simulink model "trajectory_optimization"  (R2014a)
settings: Solver=FixedStepDiscrete  StartTime=0.0  StopTime=inf  FixedStep=sample_time  RelTol=1e-3
undefined symbols (not defined in the file): alpha_apex, boom_mount_angle, control_start_time, d_y_boom_com_offset, d_y_boom_hip_offset, d_y_com, d_y_mount_to_com, DiscIntNeverNeededParam, g, h_boom, i_limit_lateral, j_segments, kd_angle, kd_lateral, kd_length, kd_motor, ki_lateral, kp_angle, kp_lateral, kp_length, kp_motor, l0_virtual, l_boom, l_boom_projected, l_retract_swing, l_seg, lateral_offset, m_leg_motor, magnitude, max_back_bar_angle, max_front_bar_angle, max_leg_angle, max_leg_length, max_torque_lateral, min_back_bar_angle, min_front_bar_angle, min_leg_angle, min_leg_length, reset_leg_angle, reset_leg_length, run_trajectory, sample_time, sea_coulomb_friction, sea_offset_friction, secondary_to_apex_target, time_to_apex, velocity_avg_samples
libraries: simulink x5
(part 1 of 2)
settings Model: xpc_rtwmakecfg_data=_xpcethercatlib_  BufferReuse=off  Creator=wmartin  LastModifiedBy=wmartin
settings SolverCC: EnableConcurrentExecution=on
settings DataIOCC: MaxDataPoints=1000000000  SaveFormat=StructureWithTime
settings OptimizationCC: BlockReduction=off  OptimizeBlockIOStorage=off  BufferReuse=off  GlobalBufferReuse=off  ExpressionFolding=off  ExpressionDepthLimit=2147483647  LocalBlockOutputs=off  SimCompilerOptimization=On
settings DebuggingCC: UnderspecifiedInitializationDetection=Classic  StateNameClashWarn=warning
settings HardwareCC: ProdIntDivRoundTo=Zero  ProdEndianess=LittleEndian  ProdHWDeviceType=Generic->32-bit x86 compatible
settings ModelReferenceCC: UpdateModelReferenceTargets=IfOutOfDate  EnableParallelModelReferenceBuilds=on  ParallelModelReferenceMATLABWorkerInit=Copy Base Workspace
settings RTWCC: SystemTargetFile=slrt.tlc  TemplateMakefile=slrt_default_tmf  Description=Simulink Real-Time  RTWVerbose=off  ProcessScript=slrt_make_rtw_hook  RTWCompilerOptimization=On
settings CodeAppCC: MaxIdLength=127
settings SimulinkRealTimeCC: GeneratePreprocessorConditionals=Disable all  EnableShiftOperators=on  RL32LogBufSizeModifier=100000000

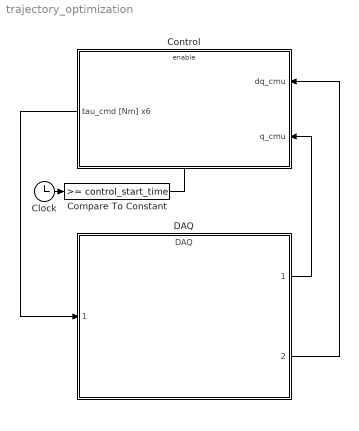
== system trajectory_optimization ==
  Clock : Clock
  Compare To Constant : simulink/Logic and Bit Operations/Compare To Constant  relop=>=  const=control_start_time  OutDataTypeStr=boolean
  Control : Subsystem
  DAQ : ModelReference  ModelNameDialog=DAQ  SimulationMode=Normal  ModelReferenceVersion=1.1653  CopyOfModelName=DAQ  DefaultDataLogging=on
  wires:
  DAQ/1 -> Control/2(q_cmu)
  DAQ/2 -> Control/1(dq_cmu)
  Clock/1 -> Compare To Constant/1
  Compare To Constant/1 -> Control/Enable
  Control/1(tau_cmd [Nm] x6) -> DAQ/1

== system trajectory_optimization/Control ==
  dq_cmu : Inport
  q_cmu : Inport  Port=2
  Enable : EnablePort  StatesWhenEnabling=reset
  Actuator Control : ModelReference  ModelNameDialog=Actuator_Control  SimulationMode=Normal  ModelReferenceVersion=1.16  CopyOfModelName=Actuator_Control  DefaultDataLogging=on
  Behavior Control : Subsystem
  Disable SEA Control : Constant  Value=[0 0 0 0]  OutDataTypeStr=boolean
  tau_cmd [Nm] x6 : Outport  InitialOutput=[0 0 0 0 0 0]
  wires:
  Behavior Control/1(motor_torque_cmd) -> Actuator Control/1
  dq_cmu/1 -> Actuator Control/4, Behavior Control/1(dq_cmu)
  Actuator Control/1 -> tau_cmd [Nm] x6/1
  q_cmu/1 -> Actuator Control/3, Behavior Control/2(q_cmu)
  Disable SEA Control/1 -> Actuator Control/2

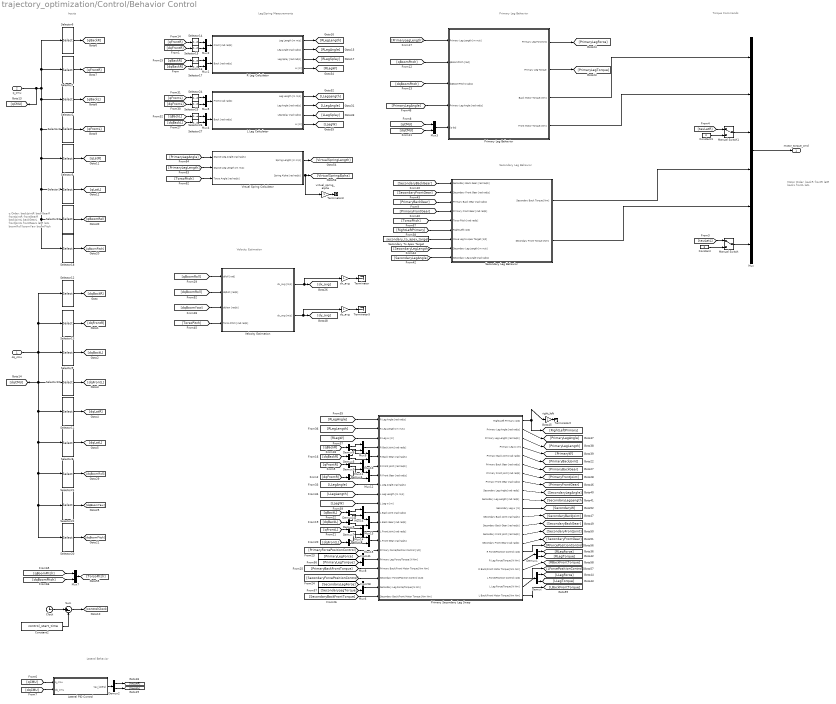
== system trajectory_optimization/Control/Behavior Control ==
  note: Motor Order:
      |
      | backR
      | frontR
      | latR
      | backL
      | frontL
      | latL
  note: q Order:
      |
      | backJointR
      | backGearR
      | frontJointR
      | frontGearR
      |
      | backJointL
      | backGearL
      | frontJointL
      | frontGearL
      |
      | latR
      | latL
      |
      | boomRoll
      | boomYaw
      | boomPitch
  note: Inputs
  note: Primary Leg Behavior
  note: Secondary Leg Behavior
  note: Torque Commands
  note: Lateral Behavior
  note: Leg/Spring Measurements
  note: Velocity Estimation
  dq_cmu : Inport
  q_cmu : Inport  Port=2
  Clock : Clock
  Constant : Constant  Value=0
  Constant1 : Constant  Value=0
  Constant2 : Constant  Value=control_start_time
  Demux{,1..10} (11 alike) : Demux  Outputs=2
  L Leg Calculator : Subsystem
  Lateral PID Control : Subsystem
  Manual Switch : ManualSwitch
  Manual Switch1 : ManualSwitch
  Mux : Mux  Inputs=6
  Mux{1..16} (16 alike) : Mux  Inputs=2
  Primary Leg Behavior : Subsystem
  Primary Secondary Leg Swap : Subsystem
  R Leg Calculator : Subsystem
  Secondary Leg Behavior : Subsystem
  Secondary To Apex Target : Constant  Value=secondary_to_apex_target  OutDataTypeStr=boolean
  Selector1 : Selector  InputPortWidth=13  Indices=[10]
  Selector10 : Selector  InputPortWidth=13  Indices=[7 8]
  Selector11 : Selector  InputPortWidth=13  Indices=[9]
  Selector12 : Selector  InputPortWidth=13  Indices=[1 2]
  Selector13 : Selector  InputPortWidth=13  Indices=[3 4]
  Selector{14..17,24..27} (8 alike) : Selector  InputPortWidth=2  Indices=[1]
  Selector18 : Selector  InputPortWidth=13  Indices=[13]
  Selector2 : Selector  InputPortWidth=13  Indices=[5 6]
  Selector20 : Selector  InputPortWidth=13  Indices=[13]
  Selector21 : Selector  InputPortWidth=13  Indices=[11]
  Selector22 : Selector  InputPortWidth=13  Indices=[12]
  Selector23 : Selector  InputPortWidth=13  Indices=[11]
  Selector4 : Selector  InputPortWidth=13  Indices=[7 8]
  Selector5 : Selector  InputPortWidth=13  Indices=[9]
  Selector6 : Selector  InputPortWidth=13  Indices=[1 2]
  Selector7 : Selector  InputPortWidth=13  Indices=[3 4]
  Selector8 : Selector  InputPortWidth=13  Indices=[10]
  Selector9 : Selector  InputPortWidth=13  Indices=[5 6]
  Sum : Sum  Inputs=|+-
  Terminator{,2..3,5} (4 alike) : Terminator
  Velocity Estimation : Subsystem
  Virtual Spring Calculator : Subsystem
  dx_avg : Gain
  dy_avg : Gain
  right_left : Gain
  virtual_spring_alpha : Gain
  motor_torque_cmd : Outport  OutputWhenDisabled=reset  InitialOutput=[0 0 0 0 0 0]
  wires:
  Lateral PID Control/1(tau_lateral) -> Demux2/1
  [dqCMU] -> Lateral PID Control/2(dq_cmu)
  [qCMU] -> Lateral PID Control/1(q_cmu)
  Sum/1 -> [controlClock]
  Selector4/1 -> [qFrontL]
  Selector2/1 -> [qBackL]
  Selector7/1 -> [qFrontR]
  Selector6/1 -> [qBackR]
  Selector1/1 -> [qLatL]
  Selector5/1 -> [qLatR]
  Constant2/1 -> Sum/2
  Clock/1 -> Sum/1
  Constant1/1 -> Manual Switch1/2
  Constant/1 -> Manual Switch/2
  Manual Switch/1 -> Mux/6
  Manual Switch1/1 -> Mux/3
  Mux/1 -> motor_torque_cmd/1
  Selector8/1 -> [dqLatL]
  Selector11/1 -> [dqLatR]
  Selector12/1 -> [dqBackR]
  Selector13/1 -> [dqFrontR]
  Selector9/1 -> [dqBackL]
  Selector10/1 -> [dqFrontL]
  [qBackR] -> Selector16/1
  [dqBackR] -> Selector17/1
  [qFrontR] -> Selector14/1
  [dqFrontR] -> Selector15/1
  Mux2/1 -> R Leg Calculator/1(Front [rad rad/s])
  Mux1/1 -> R Leg Calculator/2(Back [rad rad/s])
  R Leg Calculator/1("Leg Length [m m/s] ") -> [RLegLength]
  R Leg Calculator/2(Leg Angle [rad rad/s]) -> [RLegAngle]
  R Leg Calculator/3(Leg Splay [rad rad/s]) -> [RLegSplay]
  Demux2/1 -> [tauLatR]
  Demux2/2 -> [tauLatL]
  [tauLatR] -> Manual Switch1/1
  [tauLatL] -> Manual Switch/1
  Selector14/1 -> Mux2/1
  Selector15/1 -> Mux2/2
  Selector17/1 -> Mux1/2
  Selector16/1 -> Mux1/1
  q_cmu/1 -> Selector6/1, Selector7/1, Selector2/1, Selector4/1, Selector5/1, Selector18/1, Selector23/1, Selector1/1, [qCMU]
  Selector18/1 -> [qBoomPitch]
  Selector20/1 -> [dqBoomPitch]
  Selector22/1 -> [dqBoomYaw]
  dq_cmu/1 -> Selector20/1, Selector22/1, Selector21/1, Selector8/1, Selector11/1, Selector10/1, [dqCMU], Selector12/1, Selector13/1, Selector9/1
  Selector21/1 -> [dqBoomRoll]
  Selector23/1 -> [qBoomRoll]
  [qBackL] -> Selector26/1
  [dqBackL] -> Selector27/1
  [qFrontL] -> Selector24/1
  [dqFrontL] -> Selector25/1
  Mux5/1 -> L Leg Calculator/1(Front [rad rad/s])
  Mux4/1 -> L Leg Calculator/2(Back [rad rad/s])
  L Leg Calculator/1("Leg Length [m m/s] ") -> [LLegLength]
  L Leg Calculator/2(Leg Angle [rad rad/s]) -> [LLegAngle]
  L Leg Calculator/3(Leg Splay [rad rad/s]) -> [LLegSplay]
  Selector24/1 -> Mux5/1
  Selector25/1 -> Mux5/2
  Selector27/1 -> Mux4/2
  Selector26/1 -> Mux4/1
  R Leg Calculator/4(w [m]) -> [RLegW]
  L Leg Calculator/4(w [m]) -> [LLegW]
  Primary Secondary Leg Swap/1(Right/Left Primary [1/0]) -> right_left/1, [RightLeftPrimary]
  [PrimaryLegLength] -> Primary Leg Behavior/1(Primary Leg Length [m m/s])
  [qBoomPitch] -> Primary Leg Behavior/2(qBoomPitch [rad])
  [dqBoomPitch] -> Primary Leg Behavior/3(dqBoomPitch [rad/s])
  Primary Leg Behavior/1(Primary Leg Force [N]) -> [PrimaryLegForce]
  Primary Leg Behavior/2(Primary Leg Torque) -> [PrimaryLegTorque]
  Velocity Estimation/1(dx_avg [m/s]) -> dx_avg/1, [dx_avg]
  [qBoomRoll] -> Velocity Estimation/1(qRoll [rad])
  [dqBoomYaw] -> Velocity Estimation/3(dqYaw [rad/s])
  dx_avg/1 -> Terminator/1
  [PrimaryBackGear] -> Secondary Leg Behavior/3(Primary Back Gear [rad rad/s])
  [SecondaryBackGear] -> Secondary Leg Behavior/1(Secondary Back Gear [rad rad/s])
  [SecondaryFrontGear] -> Secondary Leg Behavior/2(Secondary Front Gear [rad rad/s])
  right_left/1 -> Terminator2/1
  Velocity Estimation/2(dy_avg [m/s]) -> dy_avg/1, [dy_avg]
  dy_avg/1 -> Terminator5/1
  [dqBoomRoll] -> Velocity Estimation/2(dqRoll [rad/s])
  [PrimaryLegAngle] -> Virtual Spring Calculator/1("Stance Leg Angle [rad rad/s] ")
  [PrimaryLegLength] -> Virtual Spring Calculator/2(Stance Leg Length [m m/s])
  Virtual Spring Calculator/1(Spring Length [m m/s]) -> [VirtualSpringLength]
  [TorsoPitch] -> Virtual Spring Calculator/3(Torso Angle [rad rad/s])
  Virtual Spring Calculator/2(Spring Alpha [rad rad/s]) -> virtual_spring_alpha/1, [VirtualSpringAlpha]
  [qBoomPitch] -> Mux7/1
  [dqBoomPitch] -> Mux7/2
  Mux7/1 -> [TorsoPitch]
  [TorsoPitch] -> Secondary Leg Behavior/5(Torso Pitch [rad rad/s])
  [TorsoPitch] -> Velocity Estimation/4(Torso Pitch [rad rad/s])
  [PrimaryLegAngle] -> Primary Leg Behavior/4(Primary Leg Angle [rad rad/s])
  virtual_spring_alpha/1 -> Terminator3/1
  Primary Leg Behavior/3(Back Motor Torque [Nm]) -> Mux/1
  Primary Leg Behavior/4(Front Motor Torque [Nm]) -> Mux/2
  [qCMU] -> Mux3/1
  [dqCMU] -> Mux3/2
  Mux3/1 -> Primary Leg Behavior/5("[q dq]")
  Secondary Leg Behavior/1(Secondary Back Torque [Nm]) -> Mux/4
  Secondary Leg Behavior/2(Secondary Front Torque [Nm]) -> Mux/5
  Primary Secondary Leg Swap/2(Primary Leg Angle [rad rad/s]) -> [PrimaryLegAngle]
  Primary Secondary Leg Swap/4(Primary Leg w [m]) -> [PrimaryW]
  Primary Secondary Leg Swap/3(Primary Leg Length [rad rad/s]) -> [PrimaryLegLength]
  [RLegAngle] -> Primary Secondary Leg Swap/1(R Leg Angle [rad rad/s])
  [RLegLength] -> Primary Secondary Leg Swap/2(R Leg Length [m m/s])
  [RLegW] -> Primary Secondary Leg Swap/3(R Leg w [m])
  [LLegAngle] -> Primary Secondary Leg Swap/8(L Leg Angle [rad rad/s])
  [LLegLength] -> Primary Secondary Leg Swap/9(L Leg Length [m m/s])
  [LLegW] -> Primary Secondary Leg Swap/10(L Leg w [m])
  [SecondaryLegForce] -> Mux6/1
  [SecondaryLegTorque] -> Mux6/2
  Mux6/1 -> Primary Secondary Leg Swap/19(Secondary Leg Force/Torque [N Nm])
  Mux8/1 -> Primary Secondary Leg Swap/16(Primary Leg Force/Torque [N Nm])
  [PrimaryLegTorque] -> Mux8/2
  [PrimaryLegForce] -> Mux8/1
  Primary Secondary Leg Swap/10(Secondary Leg Length [rad rad/s]) -> [SecondaryLegLength]
  Primary Secondary Leg Swap/9(Secondary Leg Angle [rad rad/s]) -> [SecondaryLegAngle]
  Primary Secondary Leg Swap/20(L Leg Force/Torque [N Nm]) -> Demux/1
  Demux/1 -> [LLegForce]
  Demux/2 -> [LLegTorque]
  Primary Secondary Leg Swap/17(R Leg Force/Torque [N Nm]) -> Demux1/1
  Demux1/1 -> [RLegForce]
  Demux1/2 -> [RLegTorque]
  [qFrontR] -> Demux3/1
  [dqFrontR] -> Demux4/1
  Mux9/1 -> Primary Secondary Leg Swap/4(R Back Joint [rad rad/s])
  Mux10/1 -> Primary Secondary Leg Swap/5(R Back Gear [rad rad/s])
  Mux11/1 -> Primary Secondary Leg Swap/6(R Front Joint [rad rad/s])
  Mux12/1 -> Primary Secondary Leg Swap/7(R Front Gear [rad rad/s])
  Demux3/1 -> Mux11/1
  Demux3/2 -> Mux12/1
  Demux4/1 -> Mux11/2
  Demux4/2 -> Mux12/2
  [dqBackR] -> Demux5/1
  [qBackR] -> Demux6/1
  Demux6/1 -> Mux9/1
  Demux6/2 -> Mux10/1
  Demux5/1 -> Mux9/2
  Demux5/2 -> Mux10/2
  [qFrontL] -> Demux7/1
  [dqFrontL] -> Demux8/1
  Mux16/1 -> Primary Secondary Leg Swap/11(L Back Joint [rad rad/s])
  Mux13/1 -> Primary Secondary Leg Swap/12(L Back Gear [rad rad/s])
  Mux14/1 -> Primary Secondary Leg Swap/13(L Front Joint [rad rad/s])
  Mux15/1 -> Primary Secondary Leg Swap/14(L Front Gear [rad rad/s])
  Demux7/1 -> Mux14/1
  Demux7/2 -> Mux15/1
  Demux8/1 -> Mux14/2
  Demux8/2 -> Mux15/2
  [dqBackL] -> Demux9/1
  [qBackL] -> Demux10/1
  Demux10/1 -> Mux16/1
  Demux10/2 -> Mux13/1
  Demux9/1 -> Mux16/2
  Demux9/2 -> Mux13/2
  [PrimaryForcePositionControl] -> Primary Secondary Leg Swap/15(Primary Force/Position Control [1/0])
  [SecondaryForcePositionControl] -> Primary Secondary Leg Swap/18(Secondary Force/Position Control [1/0])
  [PrimaryBackFrontTorque] -> Primary Secondary Leg Swap/17(Primary Back/Front Motor Torque [Nm Nm])
  [SecondaryBackFrontTorque] -> Primary Secondary Leg Swap/20(Secondary Back/Front Motor Torque [Nm Nm])
  Primary Secondary Leg Swap/5(Primary Back Joint [rad rad/s]) -> [PrimaryBackJoint]
  Primary Secondary Leg Swap/6(Primary Back Gear [rad rad/s]) -> [PrimaryBackGear]
  Primary Secondary Leg Swap/7(Primary Front Joint [rad rad/s]) -> [PrimaryFrontJoint]
  Primary Secondary Leg Swap/8(Primary Front Gear [rad rad/s]) -> [PrimaryFrontGear]
  Primary Secondary Leg Swap/12(Secondary Back Joint [rad rad/s]) -> [SecondaryBackJoint]
  Primary Secondary Leg Swap/13(Secondary Back Gear [rad rad/s]) -> [SecondaryBackGear]
  Primary Secondary Leg Swap/14(Secondary Front Joint [rad rad/s]) -> [SecondaryFrontJoint]
  Primary Secondary Leg Swap/15(Secondary Front Gear [rad rad/s]) -> [SecondaryFrontGear]
  Primary Secondary Leg Swap/11(Secondary Leg w [m]) -> [SecondaryW]
  Primary Secondary Leg Swap/19(L Force/Position Control [1/0]) -> [LForcePositionControl]
  Primary Secondary Leg Swap/16(R Force/Position Control [1/0]) -> [RForcePositionControl]
  Primary Secondary Leg Swap/18(R Back/Front Motor Torque [Nm Nm]) -> [RBackFrontTorque]
  Primary Secondary Leg Swap/21(L Back/Front Motor Torque [Nm Nm]) -> [LBackFrontTorque]
  [RightLeftPrimary] -> Secondary Leg Behavior/6(Right/Left [1/0])
  [PrimaryFrontGear] -> Secondary Leg Behavior/4(Primary Front Gear [rad rad/s])
  [SecondaryLegAngle] -> Secondary Leg Behavior/9(Secondary Leg Angle [rad rad/s])
  [SecondaryLegLength] -> Secondary Leg Behavior/8(Secondary Leg Length [m m/s])
  Secondary To Apex Target/1 -> Secondary Leg Behavior/7(Move Leg to Apex Target [1/0])

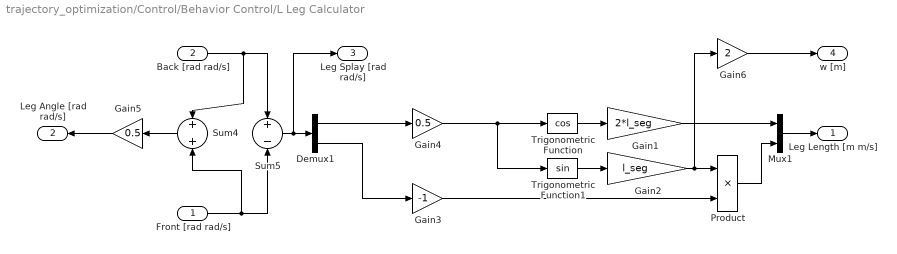
== system trajectory_optimization/Control/Behavior Control/L Leg Calculator ==
  Front [rad rad/s] : Inport
  Back [rad rad/s] : Inport  Port=2
  Demux1 : Demux  Outputs=2
  Gain1 : Gain  Gain=2*l_seg
  Gain2 : Gain  Gain=l_seg
  Gain3 : Gain  Gain=-1
  Gain4 : Gain  Gain=0.5
  Gain5 : Gain  Gain=0.5
  Gain6 : Gain  Gain=2
  Mux1 : Mux  Inputs=2
  Product : Product  RndMeth=Zero
  Sum4 : Sum  Inputs=+|+
  Sum5 : Sum  Inputs=+|-
  Trigonometric Function : Trigonometry  Operator=cos
  Trigonometric Function1 : Trigonometry
  "Leg Length [m m/s] " : Outport
  Leg Angle [rad rad/s] : Outport  Port=2
  Leg Splay [rad rad/s] : Outport  Port=3
  w [m] : Outport  Port=4
  wires:
  Gain5/1 -> Leg Angle [rad rad/s]/1
  Sum4/1 -> Gain5/1
  Mux1/1 -> "Leg Length [m m/s] "/1
  Sum5/1 -> Demux1/1, Leg Splay [rad rad/s]/1
  Gain2/1 -> Gain6/1, Product/1
  Demux1/1 -> Gain4/1
  Gain3/1 -> Product/2
  Demux1/2 -> Gain3/1
  Back [rad rad/s]/1 -> Sum5/1, Sum4/1
  Front [rad rad/s]/1 -> Sum4/2, Sum5/2
  Product/1 -> Mux1/2
  Trigonometric Function1/1 -> Gain2/1
  Gain1/1 -> Mux1/1
  Trigonometric Function/1 -> Gain1/1
  Gain4/1 -> Trigonometric Function/1, Trigonometric Function1/1
  Gain6/1 -> w [m]/1

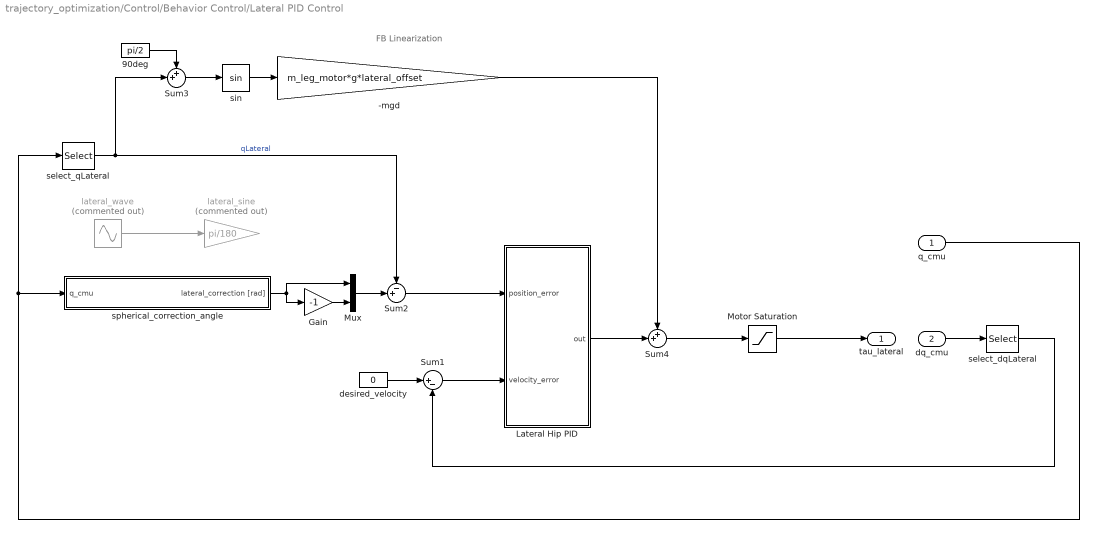
== system trajectory_optimization/Control/Behavior Control/Lateral PID Control ==
  note: FB Linearization
  q_cmu : Inport
  dq_cmu : Inport  Port=2
  -mgd : Gain  Gain=m_leg_motor*g*lateral_offset
  90deg : Constant  Value=pi/2
  Gain : Gain  Gain=-1
  Lateral Hip PID : Subsystem
  Motor Saturation : Saturate  UpperLimit=max_torque_lateral  LowerLimit=-max_torque_lateral
      settings: AttributesFormatString=Top: %<UpperLimit>\nBottom: %<LowerLimit>
  Mux : Mux  Inputs=2
  Sum1 : Sum  Inputs=|+-
  Sum2 : Sum  Inputs=-+|
  Sum3 : Sum  Inputs=++|
  Sum4 : Sum  Inputs=++|
  desired_velocity : Constant  Value=0
  lateral_sine : Gain  Commented=on  Gain=pi/180
  lateral_wave : Sin  Commented=on  Amplitude=5  Frequency=2*pi*(1/2)  SampleTime=0
  select_dqLateral : Selector  InputPortWidth=13  Indices=[9 10]
  select_qLateral : Selector  InputPortWidth=13  Indices=[9 10]
  sin : Trigonometry
  spherical_correction_angle : Subsystem
  tau_lateral : Outport
  wires:
  lateral_wave/1 -> lateral_sine/1
  Lateral Hip PID/1(out) -> Sum4/2
  Sum2/1 -> Lateral Hip PID/1(position_error)
  q_cmu/1 -> spherical_correction_angle/1(q_cmu), select_qLateral/1
  select_dqLateral/1 -> Sum1/2
  dq_cmu/1 -> select_dqLateral/1
  Sum4/1 -> Motor Saturation/1
  desired_velocity/1 -> Sum1/1
  Sum1/1 -> Lateral Hip PID/2(velocity_error)
  Gain/1 -> Mux/2
  Mux/1 -> Sum2/2
  select_qLateral/1 -> Sum3/2, Sum2/1  "qLateral"
  Motor Saturation/1 -> tau_lateral/1
  spherical_correction_angle/1(lateral_correction [rad]) -> Mux/1, Gain/1
  -mgd/1 -> Sum4/1
  Sum3/1 -> sin/1
  90deg/1 -> Sum3/1
  sin/1 -> -mgd/1

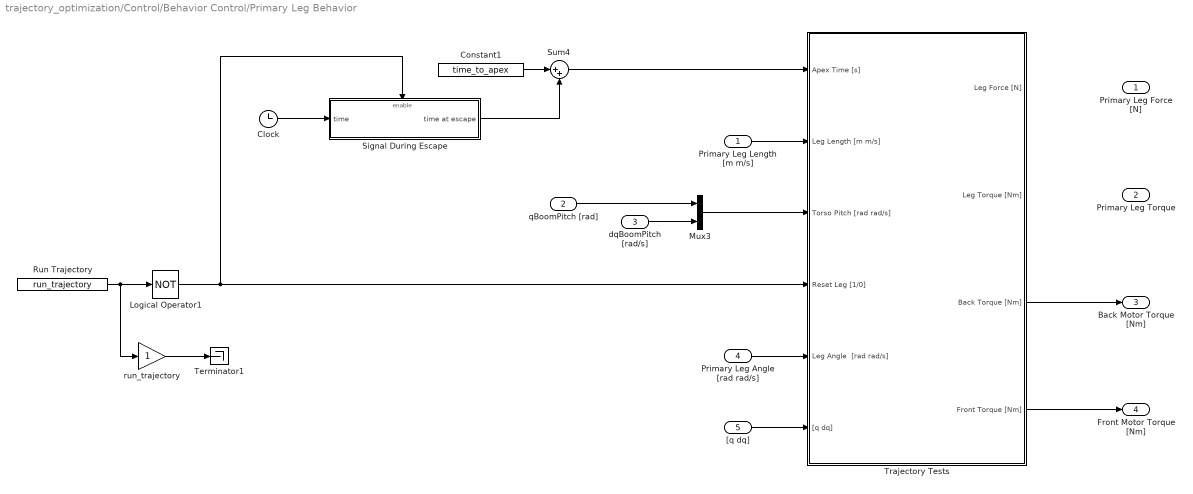
== system trajectory_optimization/Control/Behavior Control/Primary Leg Behavior ==
  Primary Leg Length [m m/s] : Inport
  qBoomPitch [rad] : Inport  Port=2
  dqBoomPitch [rad/s] : Inport  Port=3
  Primary Leg Angle [rad rad/s] : Inport  Port=4
  "[q dq]" : Inport  Port=5
  Clock : Clock
  Constant1 : Constant  Value=time_to_apex  SampleTime=sample_time
  Logical Operator1 : Logic  Operator=NOT  AllPortsSameDT=off  OutDataTypeStr=boolean
  Mux3 : Mux  Inputs=2
  Run Trajectory : Constant  Value=run_trajectory  OutDataTypeStr=boolean  SampleTime=sample_time
  Signal During Escape : Subsystem
  Sum4 : Sum  Inputs=|++
  Terminator1 : Terminator
  Trajectory Tests : Subsystem
  run_trajectory : Gain
  Primary Leg Force [N] : Outport
  Primary Leg Torque : Outport  Port=2
  Back Motor Torque [Nm] : Outport  Port=3
  Front Motor Torque [Nm] : Outport  Port=4
  wires:
  Mux3/1 -> Trajectory Tests/3(Torso Pitch [rad rad/s])
  qBoomPitch [rad]/1 -> Mux3/1
  dqBoomPitch [rad/s]/1 -> Mux3/2
  Primary Leg Length [m m/s]/1 -> Trajectory Tests/2(Leg Length [m m/s])
  Sum4/1 -> Trajectory Tests/1(Apex Time [s])
  Signal During Escape/1(time at escape) -> Sum4/2
  Clock/1 -> Signal During Escape/1(time)
  Constant1/1 -> Sum4/1
  Primary Leg Angle [rad rad/s]/1 -> Trajectory Tests/5(Leg Angle  [rad rad/s])
  Run Trajectory/1 -> run_trajectory/1, Logical Operator1/1
  Logical Operator1/1 -> Signal During Escape/Enable, Trajectory Tests/4(Reset Leg [1/0])
  Trajectory Tests/4(Front Torque [Nm]) -> Front Motor Torque [Nm]/1
  Trajectory Tests/3(Back Torque [Nm]) -> Back Motor Torque [Nm]/1
  "[q dq]"/1 -> Trajectory Tests/6("[q dq]")
  run_trajectory/1 -> Terminator1/1

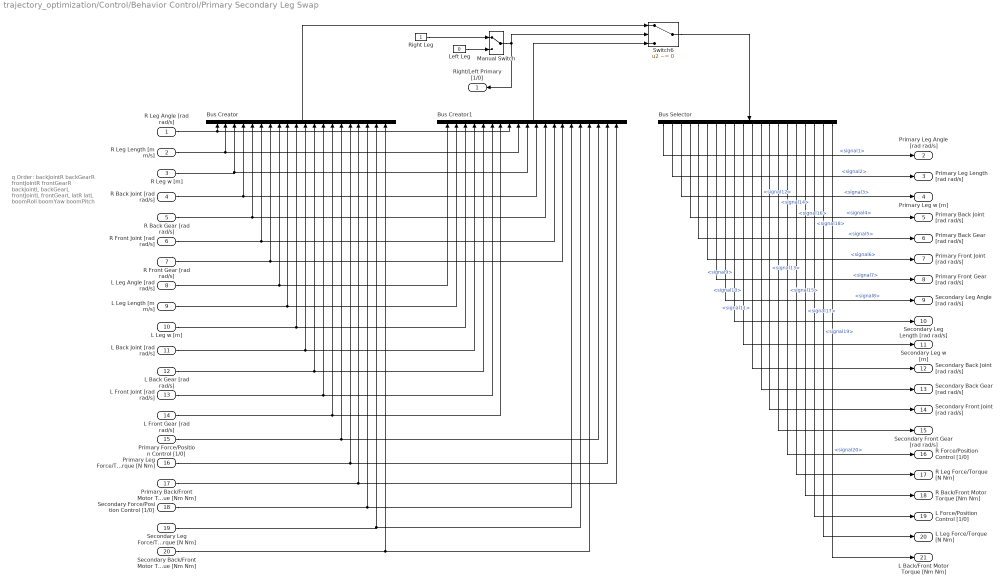
== system trajectory_optimization/Control/Behavior Control/Primary Secondary Leg Swap ==
  note: q Order:
      |
      | backJointR
      | backGearR
      | frontJointR
      | frontGearR
      |
      | backJointL
      | backGearL
      | frontJointL
      | frontGearL
      |
      | latR
      | latL
      |
      | boomRoll
      | boomYaw
      | boomPitch
  R Leg Angle [rad rad/s] : Inport
  R Leg Length [m m/s] : Inport  Port=2
  R Leg w [m] : Inport  Port=3
  R Back Joint [rad rad/s] : Inport  Port=4
  R Back Gear [rad rad/s] : Inport  Port=5
  R Front Joint [rad rad/s] : Inport  Port=6
  R Front Gear [rad rad/s] : Inport  Port=7
  L Leg Angle [rad rad/s] : Inport  Port=8
  L Leg Length [m m/s] : Inport  Port=9
  L Leg w [m] : Inport  Port=10
  L Back Joint [rad rad/s] : Inport  Port=11
  L Back Gear [rad rad/s] : Inport  Port=12
  L Front Joint [rad rad/s] : Inport  Port=13
  L Front Gear [rad rad/s] : Inport  Port=14
  Primary Force/Position Control [1/0] : Inport  Port=15
  Primary Leg Force/Torque [N Nm] : Inport  Port=16
  Primary Back/Front Motor Torque [Nm Nm] : Inport  Port=17
  Secondary Force/Position Control [1/0] : Inport  Port=18
  Secondary Leg Force/Torque [N Nm] : Inport  Port=19
  Secondary Back/Front Motor Torque [Nm Nm] : Inport  Port=20
  Bus Creator : BusCreator  Inputs=20
  Bus Creator1 : BusCreator  Inputs=20
  Bus Selector : BusSelector  OutputSignals=signal1,signal2,signal3,signal4,signal5,signal6,signal7,signal8,signal9,signal10,signal11,signal12,signal13,signal14,signal15,signal16,signal17,signal18,signal19,signal20
  Left Leg : Constant  Value=0  OutDataTypeStr=boolean
  Manual Switch : ManualSwitch
  Right Leg : Constant  OutDataTypeStr=boolean
  Switch6 : Switch  Criteria=u2 ~= 0  ZeroCross=off
  Right/Left Primary [1/0] : Outport
  Primary Leg Angle [rad rad/s] : Outport  Port=2
  Primary Leg Length [rad rad/s] : Outport  Port=3
  Primary Leg w [m] : Outport  Port=4
  Primary Back Joint [rad rad/s] : Outport  Port=5
  Primary Back Gear [rad rad/s] : Outport  Port=6
  Primary Front Joint [rad rad/s] : Outport  Port=7
  Primary Front Gear [rad rad/s] : Outport  Port=8
  Secondary Leg Angle [rad rad/s] : Outport  Port=9
  Secondary Leg Length [rad rad/s] : Outport  Port=10
  Secondary Leg w [m] : Outport  Port=11
  Secondary Back Joint [rad rad/s] : Outport  Port=12
  Secondary Back Gear [rad rad/s] : Outport  Port=13
  Secondary Front Joint [rad rad/s] : Outport  Port=14
  Secondary Front Gear [rad rad/s] : Outport  Port=15
  R Force/Position Control [1/0] : Outport  Port=16
  R Leg Force/Torque [N Nm] : Outport  Port=17
  R Back/Front Motor Torque [Nm Nm] : Outport  Port=18
  L Force/Position Control [1/0] : Outport  Port=19
  L Leg Force/Torque [N Nm] : Outport  Port=20
  L Back/Front Motor Torque [Nm Nm] : Outport  Port=21
  wires:
  Right Leg/1 -> Manual Switch/1
  Manual Switch/1 -> Switch6/2, Right/Left Primary [1/0]/1
  Left Leg/1 -> Manual Switch/2
  R Leg w [m]/1 -> Bus Creator1/10, Bus Creator/3
  R Leg Angle [rad rad/s]/1 -> Bus Creator1/8, Bus Creator/1
  R Leg Length [m m/s]/1 -> Bus Creator1/9, Bus Creator/2
  Bus Creator/1 -> Switch6/1
  Bus Creator1/1 -> Switch6/3
  R Back Joint [rad rad/s]/1 -> Bus Creator1/11, Bus Creator/4
  R Back Gear [rad rad/s]/1 -> Bus Creator1/12, Bus Creator/5
  R Front Joint [rad rad/s]/1 -> Bus Creator1/13, Bus Creator/6
  R Front Gear [rad rad/s]/1 -> Bus Creator1/14, Bus Creator/7
  L Leg Angle [rad rad/s]/1 -> Bus Creator1/1, Bus Creator/8
  L Leg Length [m m/s]/1 -> Bus Creator1/2, Bus Creator/9
  L Leg w [m]/1 -> Bus Creator1/3, Bus Creator/10
  L Back Joint [rad rad/s]/1 -> Bus Creator1/4, Bus Creator/11
  L Back Gear [rad rad/s]/1 -> Bus Creator1/5, Bus Creator/12
  L Front Joint [rad rad/s]/1 -> Bus Creator/13, Bus Creator1/6
  L Front Gear [rad rad/s]/1 -> Bus Creator1/7, Bus Creator/14
  Primary Force/Position Control [1/0]/1 -> Bus Creator1/18, Bus Creator/15
  Primary Leg Force/Torque [N Nm]/1 -> Bus Creator1/19, Bus Creator/16
  Primary Back/Front Motor Torque [Nm Nm]/1 -> Bus Creator1/20, Bus Creator/17
  Secondary Force/Position Control [1/0]/1 -> Bus Creator1/15, Bus Creator/18
  Secondary Leg Force/Torque [N Nm]/1 -> Bus Creator1/16, Bus Creator/19
  Secondary Back/Front Motor Torque [Nm Nm]/1 -> Bus Creator1/17, Bus Creator/20
  Switch6/1 -> Bus Selector/1
  Bus Selector/1 -> Primary Leg Angle [rad rad/s]/1  "<signal1>"
  Bus Selector/2 -> Primary Leg Length [rad rad/s]/1  "<signal2>"
  Bus Selector/3 -> Primary Leg w [m]/1  "<signal3>"
  Bus Selector/4 -> Primary Back Joint [rad rad/s]/1  "<signal4>"
  Bus Selector/5 -> Primary Back Gear [rad rad/s]/1  "<signal5>"
  Bus Selector/6 -> Primary Front Joint [rad rad/s]/1  "<signal6>"
  Bus Selector/7 -> Primary Front Gear [rad rad/s]/1  "<signal7>"
  Bus Selector/8 -> Secondary Leg Angle [rad rad/s]/1  "<signal8>"
  Bus Selector/9 -> Secondary Leg Length [rad rad/s]/1  "<signal9>"
  Bus Selector/10 -> Secondary Leg w [m]/1  "<signal10>"
  Bus Selector/11 -> Secondary Back Joint [rad rad/s]/1  "<signal11>"
  Bus Selector/12 -> Secondary Back Gear [rad rad/s]/1  "<signal12>"
  Bus Selector/13 -> Secondary Front Joint [rad rad/s]/1  "<signal13>"
  Bus Selector/14 -> Secondary Front Gear [rad rad/s]/1  "<signal14>"
  Bus Selector/15 -> R Force/Position Control [1/0]/1  "<signal15>"
  Bus Selector/16 -> R Leg Force/Torque [N Nm]/1  "<signal16>"
  Bus Selector/17 -> R Back/Front Motor Torque [Nm Nm]/1  "<signal17>"
  Bus Selector/18 -> L Force/Position Control [1/0]/1  "<signal18>"
  Bus Selector/19 -> L Leg Force/Torque [N Nm]/1  "<signal19>"
  Bus Selector/20 -> L Back/Front Motor Torque [Nm Nm]/1  "<signal20>"

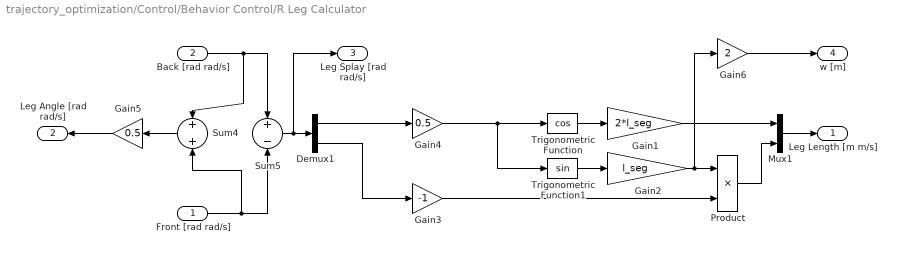
== system trajectory_optimization/Control/Behavior Control/R Leg Calculator ==
  Front [rad rad/s] : Inport
  Back [rad rad/s] : Inport  Port=2
  Demux1 : Demux  Outputs=2
  Gain1 : Gain  Gain=2*l_seg
  Gain2 : Gain  Gain=l_seg
  Gain3 : Gain  Gain=-1
  Gain4 : Gain  Gain=0.5
  Gain5 : Gain  Gain=0.5
  Gain6 : Gain  Gain=2
  Mux1 : Mux  Inputs=2
  Product : Product  RndMeth=Zero
  Sum4 : Sum  Inputs=+|+
  Sum5 : Sum  Inputs=+|-
  Trigonometric Function : Trigonometry  Operator=cos
  Trigonometric Function1 : Trigonometry
  "Leg Length [m m/s] " : Outport
  Leg Angle [rad rad/s] : Outport  Port=2
  Leg Splay [rad rad/s] : Outport  Port=3
  w [m] : Outport  Port=4
  wires:
  Gain6/1 -> w [m]/1
  Gain4/1 -> Trigonometric Function1/1, Trigonometric Function/1
  Trigonometric Function/1 -> Gain1/1
  Gain1/1 -> Mux1/1
  Trigonometric Function1/1 -> Gain2/1
  Product/1 -> Mux1/2
  Front [rad rad/s]/1 -> Sum5/2, Sum4/2
  Back [rad rad/s]/1 -> Sum4/1, Sum5/1
  Demux1/2 -> Gain3/1
  Gain3/1 -> Product/2
  Demux1/1 -> Gain4/1
  Gain2/1 -> Product/1, Gain6/1
  Sum5/1 -> Leg Splay [rad rad/s]/1, Demux1/1
  Mux1/1 -> "Leg Length [m m/s] "/1
  Sum4/1 -> Gain5/1
  Gain5/1 -> Leg Angle [rad rad/s]/1

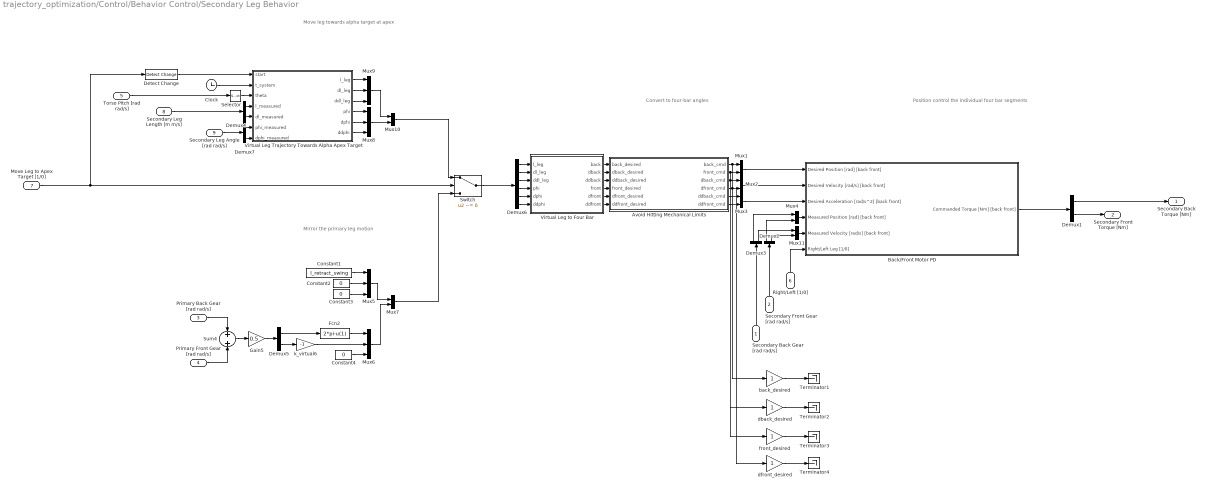
== system trajectory_optimization/Control/Behavior Control/Secondary Leg Behavior ==
  note: Mirror the primary
      | leg motion
  note: Move leg towards
      | alpha target at apex
  note: Position control the
      | individual four bar segments
  note: Convert to
      | four-bar angles
  Secondary Back Gear [rad rad/s] : Inport
  Secondary Front Gear [rad rad/s] : Inport  Port=2
  Primary Back Gear [rad rad/s] : Inport  Port=3
  Primary Front Gear [rad rad/s] : Inport  Port=4
  Torso Pitch [rad rad/s] : Inport  Port=5
  Right/Left [1/0] : Inport  Port=6
  Move Leg to Apex Target [1/0] : Inport  Port=7
  Secondary Leg Length [m m/s] : Inport  Port=8
  Secondary Leg Angle [rad rad/s] : Inport  Port=9
  Avoid Hitting Mechanical Limits : MATLAB Function  TreatAsAtomicUnit=on
  Back/Front Motor PD : Subsystem
  Clock : Clock
  Constant1 : Constant  Value=l_retract_swing
  Constant2 : Constant  Value=0
  Constant3 : Constant  Value=0
  Constant4 : Constant  Value=0
  Demux{1..5,7} (6 alike) : Demux  Outputs=2
  Demux6 : Demux  Outputs=6
  Detect Change : simulink/Logic and Bit Operations/Detect Change  vinit=0  InputProcessing=Inherited  OutDataTypeStr=boolean
  Fcn2 : Fcn  Expr=2*pi-u(1)
  Gain5 : Gain  Gain=0.5
  Mux{1..4,7,10..11} (7 alike) : Mux  Inputs=2
  Mux{5..6,8..9} (4 alike) : Mux  Inputs=3
  Selector : Selector  InputPortWidth=2  Indices=[1]
  Sum4 : Sum  Inputs=+|+
  Switch : Switch  Criteria=u2 ~= 0
  Terminator{1..4} (4 alike) : Terminator
  Virtual Leg Trajectory Towards Alpha Apex Target : MATLAB Function  TreatAsAtomicUnit=on
  Virtual Leg to Four Bar : MATLAB Function  TreatAsAtomicUnit=on
  back_desired : Gain
  dback_desired : Gain
  dfront_desired : Gain
  front_desired : Gain
  k_virtual6 : Gain  Gain=-1
  Secondary Back Torque [Nm] : Outport
  Secondary Front Torque [Nm] : Outport  Port=2
  wires:
  Demux5/2 -> k_virtual6/1
  Demux5/1 -> Fcn2/1
  Back/Front Motor PD/1(Commanded Torque [Nm] [back front]) -> Demux1/1
  Demux1/1 -> Secondary Back Torque [Nm]/1
  Demux1/2 -> Secondary Front Torque [Nm]/1
  Sum4/1 -> Gain5/1
  Primary Back Gear [rad rad/s]/1 -> Sum4/1
  Primary Front Gear [rad rad/s]/1 -> Sum4/2
  Gain5/1 -> Demux5/1
  Constant2/1 -> Mux5/2
  Constant3/1 -> Mux5/3
  Constant1/1 -> Mux5/1
  Constant4/1 -> Mux6/3
  k_virtual6/1 -> Mux6/2
  Fcn2/1 -> Mux6/1
  Move Leg to Apex Target [1/0]/1 -> Detect Change/1, Switch/2
  Mux7/1 -> Switch/3
  Switch/1 -> Demux6/1
  Mux9/1 -> Mux10/1
  Mux8/1 -> Mux10/2
  Mux10/1 -> Switch/1
  Torso Pitch [rad rad/s]/1 -> Selector/1
  Selector/1 -> Virtual Leg Trajectory Towards Alpha Apex Target/3(theta)
  Mux5/1 -> Mux7/1
  Mux6/1 -> Mux7/2
  Virtual Leg Trajectory Towards Alpha Apex Target/6(ddphi) -> Mux8/3
  Virtual Leg Trajectory Towards Alpha Apex Target/5(dphi) -> Mux8/2
  Virtual Leg Trajectory Towards Alpha Apex Target/4(phi) -> Mux8/1
  Virtual Leg Trajectory Towards Alpha Apex Target/3(ddl_leg) -> Mux9/3
  Virtual Leg Trajectory Towards Alpha Apex Target/2(dl_leg) -> Mux9/2
  Virtual Leg Trajectory Towards Alpha Apex Target/1(l_leg) -> Mux9/1
  Detect Change/1 -> Virtual Leg Trajectory Towards Alpha Apex Target/1(start)
  Clock/1 -> Virtual Leg Trajectory Towards Alpha Apex Target/2(t_system)
  Demux4/2 -> Virtual Leg Trajectory Towards Alpha Apex Target/5(dl_measured)
  Demux4/1 -> Virtual Leg Trajectory Towards Alpha Apex Target/4(l_measured)
  Demux7/1 -> Virtual Leg Trajectory Towards Alpha Apex Target/6(phi_measured)
  Demux7/2 -> Virtual Leg Trajectory Towards Alpha Apex Target/7(dphi_measured)
  Secondary Leg Length [m m/s]/1 -> Demux4/1
  Secondary Leg Angle [rad rad/s]/1 -> Demux7/1
  Virtual Leg to Four Bar/1(back) -> Avoid Hitting Mechanical Limits/1(back_desired)
  Virtual Leg to Four Bar/2(dback) -> Avoid Hitting Mechanical Limits/2(dback_desired)
  Virtual Leg to Four Bar/3(ddback) -> Avoid Hitting Mechanical Limits/3(ddback_desired)
  Virtual Leg to Four Bar/4(front) -> Avoid Hitting Mechanical Limits/4(front_desired)
  Virtual Leg to Four Bar/5(dfront) -> Avoid Hitting Mechanical Limits/5(dfront_desired)
  Virtual Leg to Four Bar/6(ddfront) -> Avoid Hitting Mechanical Limits/6(ddfront_desired)
  Demux6/1 -> Virtual Leg to Four Bar/1(l_leg)
  Demux6/2 -> Virtual Leg to Four Bar/2(dl_leg)
  Demux6/3 -> Virtual Leg to Four Bar/3(ddl_leg)
  Demux6/4 -> Virtual Leg to Four Bar/4(phi)
  Demux6/5 -> Virtual Leg to Four Bar/5(dphi)
  Demux6/6 -> Virtual Leg to Four Bar/6(ddphi)
  back_desired/1 -> Terminator1/1
  dback_desired/1 -> Terminator2/1
  front_desired/1 -> Terminator3/1
  dfront_desired/1 -> Terminator4/1
  Mux11/1 -> Back/Front Motor PD/5(Measured Velocity [rad/s] [back front])
  Demux2/2 -> Mux11/2
  Mux4/1 -> Back/Front Motor PD/4(Measured Position [rad] [back front])
  Mux1/1 -> Back/Front Motor PD/1(Desired Position [rad] [back front])
  Right/Left [1/0]/1 -> Back/Front Motor PD/6(Right/Left Leg [1/0])
  Demux3/2 -> Mux11/1
  Demux3/1 -> Mux4/1
  Avoid Hitting Mechanical Limits/2(front_cmd) -> front_desired/1, Mux1/2
  Avoid Hitting Mechanical Limits/1(back_cmd) -> back_desired/1, Mux1/1
  Demux2/1 -> Mux4/2
  Secondary Front Gear [rad rad/s]/1 -> Demux2/1
  Secondary Back Gear [rad rad/s]/1 -> Demux3/1
  Avoid Hitting Mechanical Limits/3(dback_cmd) -> dback_desired/1, Mux2/1
  Avoid Hitting Mechanical Limits/4(dfront_cmd) -> dfront_desired/1, Mux2/2
  Avoid Hitting Mechanical Limits/5(ddback_cmd) -> Mux3/1
  Avoid Hitting Mechanical Limits/6(ddfront_cmd) -> Mux3/2
  Mux2/1 -> Back/Front Motor PD/2(Desired Velocity [rad/s] [back front])
  Mux3/1 -> Back/Front Motor PD/3(Desired Acceleration [rad/s^2] [back front])

== system trajectory_optimization/Control/Behavior Control/Velocity Estimation ==
  qRoll [rad] : Inport
  dqRoll [rad/s] : Inport  Port=2
  dqYaw [rad/s] : Inport  Port=3
  Torso Pitch [rad rad/s] : Inport  Port=4
  Demux : Demux  Outputs=2
  Mux : Mux  Inputs=2
  Recursive Moving Average : Subsystem
  Selector : Selector  InputPortWidth=2  Indices=[2]
  Terminator2 : Terminator
  Terminator7 : Terminator
  dx_and_dy_from_yaw_and_roll : MATLAB Function  TreatAsAtomicUnit=on
  y_com : Gain
  y_hip : Gain
  dx_avg [m/s] : Outport
  dy_avg [m/s] : Outport  Port=2
  wires:
  Recursive Moving Average/1(Average Velocity [m/s]) -> Demux/1
  dx_and_dy_from_yaw_and_roll/1(dx) -> Mux/1
  dqYaw [rad/s]/1 -> dx_and_dy_from_yaw_and_roll/3(dqYaw)
  Selector/1 -> dx_and_dy_from_yaw_and_roll/4(dqPitch)
  dx_and_dy_from_yaw_and_roll/2(dy) -> Mux/2
  Mux/1 -> Recursive Moving Average/1(Velocity [m/s])
  Demux/1 -> dx_avg [m/s]/1
  Demux/2 -> dy_avg [m/s]/1
  Torso Pitch [rad rad/s]/1 -> Selector/1
  dqRoll [rad/s]/1 -> dx_and_dy_from_yaw_and_roll/2(dqRoll)
  qRoll [rad]/1 -> dx_and_dy_from_yaw_and_roll/1(qRoll)
  dx_and_dy_from_yaw_and_roll/3(y_com) -> y_com/1
  y_com/1 -> Terminator2/1
  y_hip/1 -> Terminator7/1
  dx_and_dy_from_yaw_and_roll/4(y_hip) -> y_hip/1

== system trajectory_optimization/Control/Behavior Control/Virtual Spring Calculator ==
  "Stance Leg Angle [rad rad/s] " : Inport
  Stance Leg Length [m m/s] : Inport  Port=2
  Torso Angle [rad rad/s] : Inport  Port=3
  Demux : Demux  Outputs=2
  Demux1 : Demux  Outputs=2
  Demux2 : Demux  Outputs=2
  Mux3 : Mux  Inputs=2
  Mux4 : Mux  Inputs=2
  Virtual Spring Calculations : MATLAB Function  TreatAsAtomicUnit=on
  Spring Length [m m/s] : Outport
  Spring Alpha [rad rad/s] : Outport  Port=2  OutDataTypeStr=double  PortDimensions=2
  wires:
  Mux4/1 -> Spring Alpha [rad rad/s]/1
  Virtual Spring Calculations/4(dl_v) -> Mux3/2
  Virtual Spring Calculations/3(l_v) -> Mux3/1
  Virtual Spring Calculations/2(dalpha_v) -> Mux4/2
  Virtual Spring Calculations/1(alpha_v) -> Mux4/1
  Demux1/2 -> Virtual Spring Calculations/4(dl)
  Demux2/2 -> Virtual Spring Calculations/6(dphi)
  Demux2/1 -> Virtual Spring Calculations/5(phi)
  Demux1/1 -> Virtual Spring Calculations/3(l)
  Demux/2 -> Virtual Spring Calculations/2(dth)
  Demux/1 -> Virtual Spring Calculations/1(th)
  Torso Angle [rad rad/s]/1 -> Demux/1
  "Stance Leg Angle [rad rad/s] "/1 -> Demux2/1
  Mux3/1 -> Spring Length [m m/s]/1
  Stance Leg Length [m m/s]/1 -> Demux1/1

== system trajectory_optimization/Control/Behavior Control/Lateral PID Control/Lateral Hip PID ==
  position_error : Inport
  velocity_error : Inport  Port=2
  Discrete-Time Integrator : DiscreteIntegrator  IntegratorMethod=Integration: Trapezoidal  SampleTime=sample_time  LimitOutput=on  UpperSaturationLimit=i_limit_lateral  LowerSaturationLimit=-i_limit_lateral  ICPrevOutput=DiscIntNeverNeededParam  ICPrevScaledInput=DiscIntNeverNeededParam
  Sum : Sum  Inputs=+++
  kd_lateral : Gain  Description=xPCTag(1)=kd_lateral;  Gain=kd_lateral
  ki_lateral : Gain  Description=xPCTag(1)=ki_lateral;  Gain=ki_lateral
  kp_lateral : Gain  Description=xPCTag(1)=kp_lateral;  Gain=kp_lateral
  out : Outport
  wires:
  velocity_error/1 -> kd_lateral/1
  Discrete-Time Integrator/1 -> Sum/3
  ki_lateral/1 -> Discrete-Time Integrator/1
  kp_lateral/1 -> Sum/2
  position_error/1 -> ki_lateral/1, kp_lateral/1
  Sum/1 -> out/1
  kd_lateral/1 -> Sum/1

== system trajectory_optimization/Control/Behavior Control/Lateral PID Control/spherical_correction_angle ==
  q_cmu : Inport
  Selector : Selector  InputPortWidth=13  Indices=[11]
  Sum1 : Sum  Inputs=|+-
  Terminator2 : Terminator
  boom_mount_angle : Constant  Value=boom_mount_angle
  lateral_correction : Gain  Gain=180/pi
  lateral_correction [rad] : Outport
  wires:
  Sum1/1 -> lateral_correction/1, lateral_correction [rad]/1
  Selector/1 -> Sum1/1  "qBoomRoll"
  q_cmu/1 -> Selector/1
  boom_mount_angle/1 -> Sum1/2
  lateral_correction/1 -> Terminator2/1

== system trajectory_optimization/Control/Behavior Control/Primary Leg Behavior/Signal During Escape ==
  time : Inport
  Enable : EnablePort
  time at escape : Outport  InitialOutput=[0]
  wires:
  time/1 -> time at escape/1

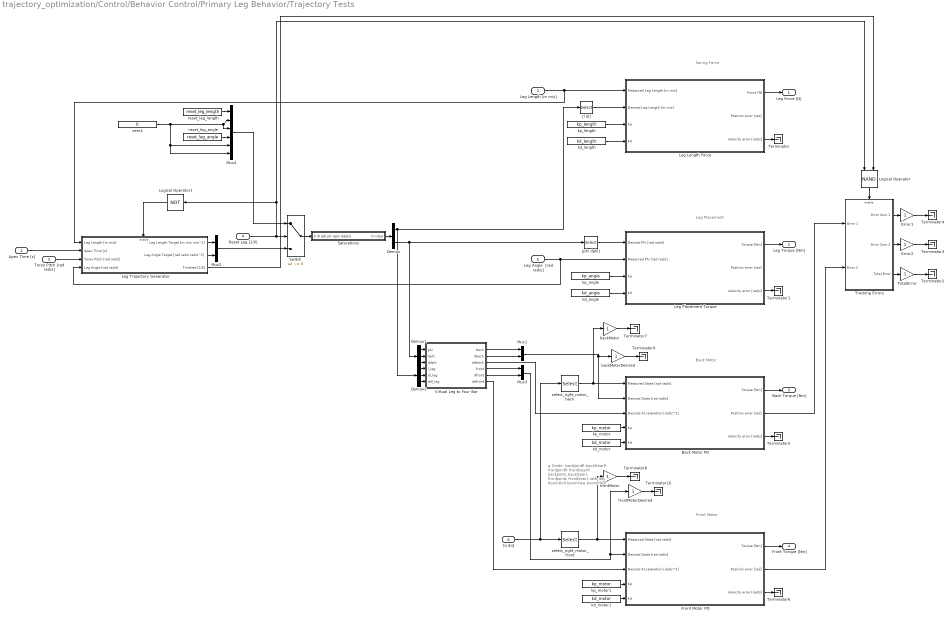
== system trajectory_optimization/Control/Behavior Control/Primary Leg Behavior/Trajectory Tests ==
  note: Leg Placement
  note: Spring Force
  note: Front Motor
  note: Back Motor
  note: q Order:
      |
      | backJointR
      | backGearR
      | frontJointR
      | frontGearR
      |
      | backJointL
      | backGearL
      | frontJointL
      | frontGearL
      |
      | latR
      | latL
      |
      | boomRoll
      | boomYaw
      | boomPitch
  Apex Time [s] : Inport
  Leg Length [m m/s] : Inport  Port=2
  Torso Pitch [rad rad/s] : Inport  Port=3
  Reset Leg [1/0] : Inport  Port=4
  Leg Angle  [rad rad/s] : Inport  Port=5
  "[q dq]" : Inport  Port=6
  Back Motor PD : Subsystem
  Demux : Demux  Outputs=2
  Demux1 : Demux  Outputs=3
  Demux2 : Demux  Outputs=3
  Error1 : Gain
  Error2 : Gain
  Front Motor PD : Subsystem
  Leg Length Force : Subsystem
  Leg Placement Torque : Subsystem
  Leg Trajectory Generator : Subsystem
  Logical Operator : Logic  Operator=NAND  IconShape=distinctive  AllPortsSameDT=off  OutDataTypeStr=boolean
  Logical Operator1 : Logic  Operator=NOT  IconShape=distinctive  AllPortsSameDT=off  OutDataTypeStr=boolean
  Mux1 : Mux  Inputs=2
  Mux2 : Mux  Inputs=2
  Mux3 : Mux  Inputs=2
  Mux4 : Mux  Inputs=6
  Saturations : Subsystem
  Switch : Switch  Criteria=u2 ~= 0
  Terminator{,1..10} (11 alike) : Terminator
  TotalError : Gain
  Tracking Errors : Subsystem
  Virtual Leg to Four Bar : MATLAB Function  TreatAsAtomicUnit=on
  "[l dl]" : Selector  InputPortWidth=3  Indices=[1 2]
  "[phi dphi]" : Selector  InputPortWidth=3  Indices=[1 2]
  backMotor : Gain
  backMotorDesired : Gain
  frontMotor : Gain
  frontMotorDesired : Gain
  kd_angle : Constant  Value=kd_angle
  kd_length : Constant  Value=kd_length
  kd_motor : Constant  Value=kd_motor
  kd_motor1 : Constant  Value=kd_motor
  kp_angle : Constant  Value=kp_angle
  kp_length : Constant  Value=kp_length
  kp_motor : Constant  Value=kp_motor
  kp_motor1 : Constant  Value=kp_motor
  reset_leg_angle : Constant  Value=reset_leg_angle  SampleTime=sample_time
  reset_leg_length : Constant  Value=reset_leg_length  SampleTime=sample_time
  select_right_motor_back : Selector  InputPortWidth=26  Indices=[2 15]
  select_right_motor_front : Selector  InputPortWidth=26  Indices=[4 17]
  zero1 : Constant  Value=0  SampleTime=sample_time
  Leg Force [N] : Outport
  Leg Torque [Nm] : Outport  Port=2
  Back Torque [Nm] : Outport  Port=3
  Front Torque [Nm] : Outport  Port=4
  wires:
  Leg Length Force/1(Force [N]) -> Leg Force [N]/1
  Leg Placement Torque/1(Torque [Nm]) -> Leg Torque [Nm]/1
  Torso Pitch [rad rad/s]/1 -> Leg Trajectory Generator/3(Torso Pitch [rad rad/s])
  Demux/2 -> "[phi dphi]"/1, Demux1/1
  Apex Time [s]/1 -> Leg Trajectory Generator/2(Apex Time [s])
  Leg Length [m m/s]/1 -> Leg Trajectory Generator/1(Leg Length [m m/s]), Leg Length Force/1(Measured Leg Length [m m/s])
  Leg Angle  [rad rad/s]/1 -> Leg Trajectory Generator/4(Leg Angle [rad rad/s]), Leg Placement Torque/2(Measured Phi [rad rad/s])
  Leg Trajectory Generator/1(Leg Length Target [m m/s m/s^2]) -> Mux2/1
  Mux2/1 -> Switch/3
  Demux/1 -> "[l dl]"/1, Demux2/1
  Switch/1 -> Saturations/1("[l dl ddl phi dphi ddphi]")
  Mux4/1 -> Switch/1
  kd_length/1 -> Leg Length Force/4(Kd)
  kp_length/1 -> Leg Length Force/3(Kp)
  kp_angle/1 -> Leg Placement Torque/3(Kp)
  kd_angle/1 -> Leg Placement Torque/4(Kd)
  Leg Length Force/3(Velocity error [rad/s]) -> Terminator/1
  Leg Placement Torque/3(Velocity error [rad/s]) -> Terminator1/1
  Tracking Errors/3(Total Error) -> TotalError/1
  TotalError/1 -> Terminator2/1
  Error2/1 -> Terminator3/1
  Tracking Errors/2(Error Sum 2) -> Error2/1
  Tracking Errors/1(Error Sum 1) -> Error1/1
  Error1/1 -> Terminator4/1
  Logical Operator/1 -> Tracking Errors/Enable
  Leg Trajectory Generator/3(Finished [1/0]) -> Logical Operator/2
  Leg Trajectory Generator/2(Leg Angle Target [rad rad/s rad/s^2]) -> Mux2/2
  Reset Leg [1/0]/1 -> Switch/2, Logical Operator1/1, Logical Operator/1
  Back Motor PD/1(Torque [Nm]) -> Back Torque [Nm]/1
  Front Motor PD/1(Torque [Nm]) -> Front Torque [Nm]/1
  kd_motor/1 -> Back Motor PD/5(Kd)
  kp_motor/1 -> Back Motor PD/4(Kp)
  Back Motor PD/3(Velocity error [rad/s]) -> Terminator5/1
  Front Motor PD/3(Velocity error [rad/s]) -> Terminator6/1
  Front Motor PD/2(Position error [rad]) -> Tracking Errors/2(Error 2)
  Back Motor PD/2(Position error [rad]) -> Tracking Errors/1(Error 1)
  kd_motor1/1 -> Front Motor PD/5(Kd)
  kp_motor1/1 -> Front Motor PD/4(Kp)
  Virtual Leg to Four Bar/2(dback) -> Mux1/2
  Virtual Leg to Four Bar/1(back) -> Mux1/1
  Virtual Leg to Four Bar/4(front) -> Mux3/1
  Virtual Leg to Four Bar/5(dfront) -> Mux3/2
  Mux1/1 -> Back Motor PD/2(Desired State [rad rad/s]), backMotorDesired/1
  "[q dq]"/1 -> select_right_motor_back/1, select_right_motor_front/1
  select_right_motor_back/1 -> Back Motor PD/1(Measured State [rad rad/s]), backMotor/1
  reset_leg_angle/1 -> Mux4/4
  reset_leg_length/1 -> Mux4/1
  zero1/1 -> Mux4/6, Mux4/5, Mux4/3, Mux4/2
  backMotor/1 -> Terminator7/1
  select_right_motor_front/1 -> frontMotor/1, Front Motor PD/1(Measured State [rad rad/s])
  frontMotor/1 -> Terminator8/1
  backMotorDesired/1 -> Terminator9/1
  Mux3/1 -> frontMotorDesired/1, Front Motor PD/2(Desired State [rad rad/s])
  frontMotorDesired/1 -> Terminator10/1
  Logical Operator1/1 -> Leg Trajectory Generator/Enable
  "[l dl]"/1 -> Leg Length Force/2(Desired Leg Length [m m/s])
  "[phi dphi]"/1 -> Leg Placement Torque/1(Desired Phi [rad rad/s])
  Demux1/1 -> Virtual Leg to Four Bar/1(phi)
  Demux1/2 -> Virtual Leg to Four Bar/2(dphi)
  Demux1/3 -> Virtual Leg to Four Bar/3(ddphi)
  Demux2/3 -> Virtual Leg to Four Bar/6(ddl_leg)
  Demux2/2 -> Virtual Leg to Four Bar/5(dl_leg)
  Demux2/1 -> Virtual Leg to Four Bar/4(l_leg)
  Virtual Leg to Four Bar/3(ddback) -> Back Motor PD/3(Desired Acceleration [rad/s^2])
  Virtual Leg to Four Bar/6(ddfront) -> Front Motor PD/3(Desired Acceleration [rad/s^2])
  Saturations/1(limited) -> Demux/1

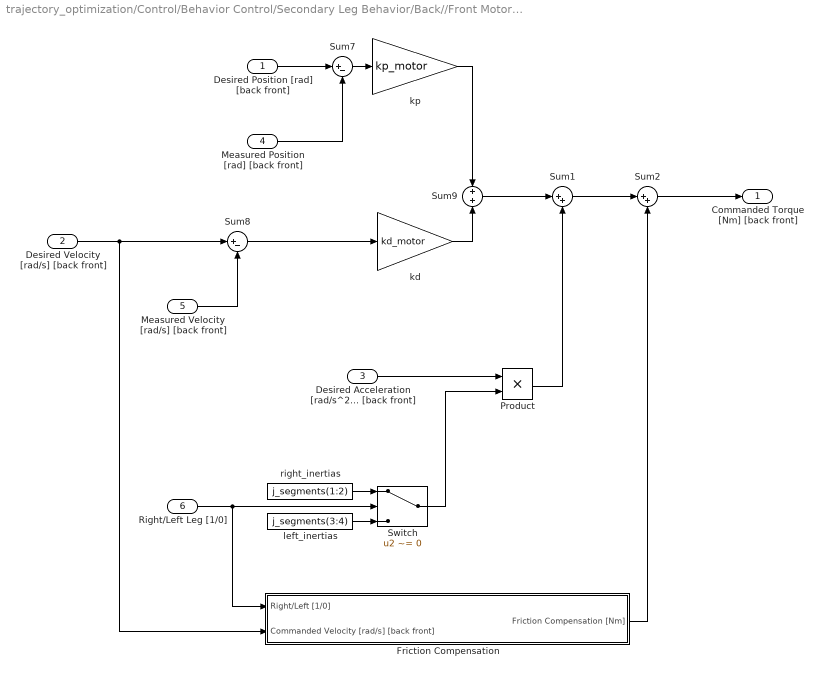
== system trajectory_optimization/Control/Behavior Control/Secondary Leg Behavior/Back//Front Motor PD ==
  Desired Position [rad] [back front] : Inport
  Desired Velocity [rad/s] [back front] : Inport  Port=2
  Desired Acceleration [rad/s^2] [back front] : Inport  Port=3
  Measured Position [rad] [back front] : Inport  Port=4
  Measured Velocity [rad/s] [back front] : Inport  Port=5
  Right/Left Leg [1/0] : Inport  Port=6
  Friction Compensation : Subsystem
  Product : Product
  Sum1 : Sum  Inputs=|++
  Sum2 : Sum  Inputs=|++
  Sum7 : Sum  Inputs=|+-
  Sum8 : Sum  Inputs=|+-
  Sum9 : Sum
  Switch : Switch  Criteria=u2 ~= 0
  kd : Gain  Gain=kd_motor
  kp : Gain  Gain=kp_motor
  left_inertias : Constant  Value=j_segments(3:4)
  right_inertias : Constant  Value=j_segments(1:2)
  Commanded Torque [Nm] [back front] : Outport
  wires:
  kp/1 -> Sum9/1
  Sum7/1 -> kp/1
  Measured Position [rad] [back front]/1 -> Sum7/2
  Sum9/1 -> Sum1/1
  Sum8/1 -> kd/1
  Desired Position [rad] [back front]/1 -> Sum7/1
  kd/1 -> Sum9/2
  Measured Velocity [rad/s] [back front]/1 -> Sum8/2
  Sum1/1 -> Sum2/1
  Desired Acceleration [rad/s^2] [back front]/1 -> Product/1
  Product/1 -> Sum1/2
  Right/Left Leg [1/0]/1 -> Friction Compensation/1(Right/Left [1/0]), Switch/2
  right_inertias/1 -> Switch/1
  left_inertias/1 -> Switch/3
  Switch/1 -> Product/2
  Sum2/1 -> Commanded Torque [Nm] [back front]/1
  Friction Compensation/1(Friction Compensation [Nm]) -> Sum2/2
  Desired Velocity [rad/s] [back front]/1 -> Friction Compensation/2(Commanded Velocity [rad/s] [back front]), Sum8/1

== system trajectory_optimization/Control/Behavior Control/Velocity Estimation/Recursive Moving Average ==
  Velocity [m/s] : Inport
  Delay : Delay  DelayLength=velocity_avg_samples  InitialCondition=0  UseCircularBuffer=on  SampleTime=sample_time
  Gain : Gain  Gain=1/velocity_avg_samples
  Sum : Sum  Inputs=-++
  Unit Delay : UnitDelay  SampleTime=sample_time
  Average Velocity [m/s] : Outport
  wires:
  Velocity [m/s]/1 -> Delay/1, Sum/2
  Sum/1 -> Unit Delay/1, Gain/1
  Delay/1 -> Sum/1
  Gain/1 -> Average Velocity [m/s]/1
  Unit Delay/1 -> Sum/3

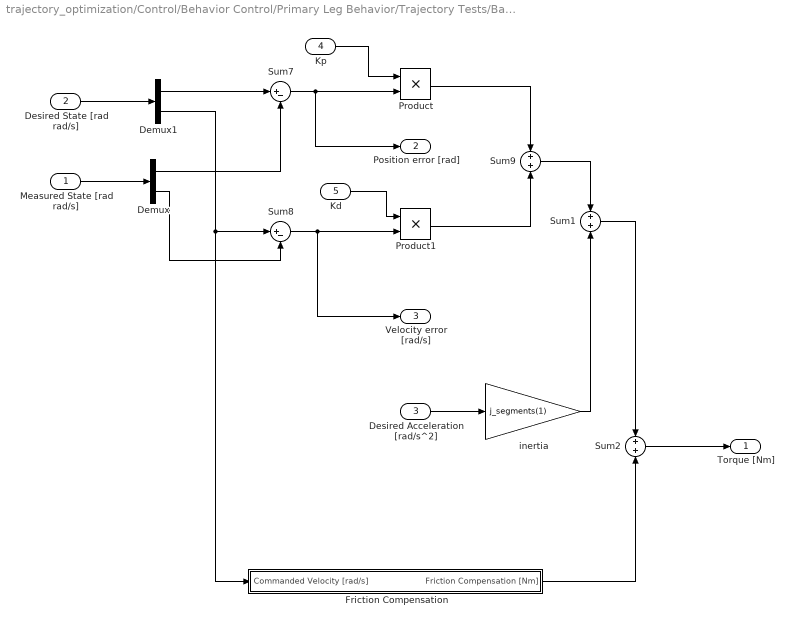
== system trajectory_optimization/Control/Behavior Control/Primary Leg Behavior/Trajectory Tests/Back Motor PD ==
  Measured State [rad rad/s] : Inport
  Desired State [rad rad/s] : Inport  Port=2
  Desired Acceleration [rad/s^2] : Inport  Port=3
  Kp : Inport  Port=4
  Kd : Inport  Port=5
  Demux : Demux  Outputs=2
  Demux1 : Demux  Outputs=2
  Friction Compensation : Subsystem
  Product : Product
  Product1 : Product
  Sum1 : Sum
  Sum2 : Sum
  Sum7 : Sum  Inputs=|+-
  Sum8 : Sum  Inputs=|+-
  Sum9 : Sum
  inertia : Gain  Gain=j_segments(1)
  Torque [Nm] : Outport  OutputWhenDisabled=reset  InitialOutput=[0]
  Position error [rad] : Outport  Port=2
  Velocity error [rad/s] : Outport  Port=3
  wires:
  Sum9/1 -> Sum1/1
  Measured State [rad rad/s]/1 -> Demux/1
  Sum7/1 -> Product/2, Position error [rad]/1
  Sum8/1 -> Product1/2, Velocity error [rad/s]/1
  Product/1 -> Sum9/1
  Demux/1 -> Sum7/2
  Demux1/2 -> Friction Compensation/1(Commanded Velocity [rad/s]), Sum8/1
  Demux1/1 -> Sum7/1
  Product1/1 -> Sum9/2
  Demux/2 -> Sum8/2
  Kp/1 -> Product/1
  Kd/1 -> Product1/1
  Desired State [rad rad/s]/1 -> Demux1/1
  Desired Acceleration [rad/s^2]/1 -> inertia/1
  inertia/1 -> Sum1/2
  Sum1/1 -> Sum2/1
  Sum2/1 -> Torque [Nm]/1
  Friction Compensation/1(Friction Compensation [Nm]) -> Sum2/2

== system trajectory_optimization/Control/Behavior Control/Primary Leg Behavior/Trajectory Tests/Front Motor PD ==
  Measured State [rad rad/s] : Inport
  Desired State [rad rad/s] : Inport  Port=2
  Desired Acceleration [rad/s^2] : Inport  Port=3
  Kp : Inport  Port=4
  Kd : Inport  Port=5
  Demux : Demux  Outputs=2
  Demux1 : Demux  Outputs=2
  Friction Compensation : Subsystem
  Product : Product
  Product1 : Product
  Sum1 : Sum
  Sum2 : Sum
  Sum7 : Sum  Inputs=|+-
  Sum8 : Sum  Inputs=|+-
  Sum9 : Sum
  inertia : Gain  Gain=j_segments(2)
  Torque [Nm] : Outport  OutputWhenDisabled=reset  InitialOutput=[0]
  Position error [rad] : Outport  Port=2
  Velocity error [rad/s] : Outport  Port=3
  wires:
  Desired State [rad rad/s]/1 -> Demux1/1
  Kd/1 -> Product1/1
  Kp/1 -> Product/1
  Demux/2 -> Sum8/2
  Product1/1 -> Sum9/2
  Demux1/1 -> Sum7/1
  Demux1/2 -> Friction Compensation/1(Commanded Velocity [rad/s]), Sum8/1
  Demux/1 -> Sum7/2
  Product/1 -> Sum9/1
  Sum8/1 -> Velocity error [rad/s]/1, Product1/2
  Sum7/1 -> Position error [rad]/1, Product/2
  Measured State [rad rad/s]/1 -> Demux/1
  Sum9/1 -> Sum2/1
  Sum1/1 -> Torque [Nm]/1
  inertia/1 -> Sum2/2
  Desired Acceleration [rad/s^2]/1 -> inertia/1
  Sum2/1 -> Sum1/1
  Friction Compensation/1(Friction Compensation [Nm]) -> Sum1/2

== system trajectory_optimization/Control/Behavior Control/Primary Leg Behavior/Trajectory Tests/Leg Length Force ==
  Measured Leg Length [m m/s] : Inport
  Desired Leg Length [m m/s] : Inport  Port=2
  Kp : Inport  Port=3
  Kd : Inport  Port=4
  Demux : Demux  Outputs=2
  Demux1 : Demux  Outputs=2
  Product : Product
  Product1 : Product
  Sum7 : Sum  Inputs=|+-
  Sum8 : Sum  Inputs=|+-
  Sum9 : Sum
  Force [N] : Outport  OutputWhenDisabled=reset  InitialOutput=[0]
  Position error [rad] : Outport  Port=2
  Velocity error [rad/s] : Outport  Port=3
  wires:
  Desired Leg Length [m m/s]/1 -> Demux1/1
  Kd/1 -> Product1/1
  Kp/1 -> Product/1
  Demux/2 -> Sum8/2
  Product1/1 -> Sum9/2
  Demux1/1 -> Sum7/1
  Demux1/2 -> Sum8/1
  Demux/1 -> Sum7/2
  Product/1 -> Sum9/1
  Sum8/1 -> Velocity error [rad/s]/1, Product1/2
  Sum7/1 -> Position error [rad]/1, Product/2
  Measured Leg Length [m m/s]/1 -> Demux/1
  Sum9/1 -> Force [N]/1

== system trajectory_optimization/Control/Behavior Control/Primary Leg Behavior/Trajectory Tests/Leg Placement Torque ==
  Desired Phi [rad rad/s] : Inport
  Measured Phi [rad rad/s] : Inport  Port=2
  Kp : Inport  Port=3
  Kd : Inport  Port=4
  Demux : Demux  Outputs=2
  Demux1 : Demux  Outputs=2
  Product : Product
  Product1 : Product
  Sum7 : Sum  Inputs=|+-
  Sum8 : Sum  Inputs=|+-
  Sum9 : Sum
  Torque [Nm] : Outport  OutputWhenDisabled=reset  InitialOutput=[0]
  Position error [rad] : Outport  Port=2
  Velocity error [rad/s] : Outport  Port=3
  wires:
  Sum9/1 -> Torque [Nm]/1
  Measured Phi [rad rad/s]/1 -> Demux/1
  Sum7/1 -> Product/2, Position error [rad]/1
  Sum8/1 -> Product1/2, Velocity error [rad/s]/1
  Product/1 -> Sum9/1
  Demux/1 -> Sum7/2
  Demux1/2 -> Sum8/1
  Demux1/1 -> Sum7/1
  Product1/1 -> Sum9/2
  Demux/2 -> Sum8/2
  Kp/1 -> Product/1
  Kd/1 -> Product1/1
  Desired Phi [rad rad/s]/1 -> Demux1/1
